simulink model "controller"  (R2017b)
settings: Solver=ode23tb  StartTime=0.0  StopTime=10  RelTol=1e-3
values from neighbouring files (symbols this model uses):
  A = [0 0 1 0 ... (first row only)    [linearizedSS.m]
  B = [0;0;K*v/alpha;-c2*l1*m2/alpha]    [linearizedSS.m]
  C = [1 0 0 0;0 1 0 0]    [linearizedSS.m]
  K = 1.8    [Nonlinearequations.m]    (also in controller.m = place(Phi',Cd',dopoles).'; controllerData2.m = place(Phi',Cd',dopoles).'; linearizedSS.m; pendulumSim.m)
  L = Laug(1:4)    [controller.m]    (also in controllerData2.m)
  x0 = [0.51*pi,0,0.5*pi,0]    [Nonlinearequations.m]    (also in controllerData3.m = [-0.6*pi 0 -0.4*pi 0]; linearizeM.m = [-0.51*pi,0,-0.5*pi,0])
settings Model: Creator=geert  LastModifiedBy=geert

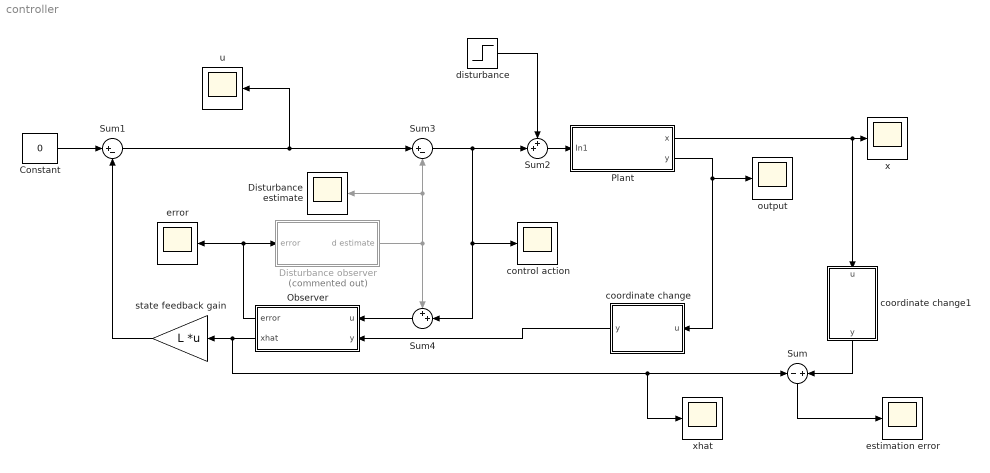
== system controller ==
  Constant : Constant  Value=0
  Disturbance estimate : Scope
  Disturbance observer : Subsystem  Commented=on
  Observer : Subsystem
  Plant : Subsystem
  Sum : Sum  Inputs=-|+
  Sum1 : Sum  Inputs=|+-
  Sum2 : Sum  Inputs=++|
  Sum3 : Sum  Inputs=|+-
  Sum4 : Sum  Inputs=++|
  control action : Scope
  coordinate change : MATLAB Function  TreatAsAtomicUnit=on
  coordinate change1 : MATLAB Function  TreatAsAtomicUnit=on
  disturbance : Step  Time=5  After=0  SampleTime=0
  error : Scope
  estimation error : Scope
  output : Scope
  state feedback gain : Gain  Gain=L  Multiplication=Matrix(K*u)
  u : Scope
  x : Scope
  xhat : Scope
  wires:
  state feedback gain/1 -> Sum1/2
  Sum2/1 -> Plant/1(In1)
  Observer/2(xhat) -> xhat/1, Sum/1, state feedback gain/1
  Sum/1 -> estimation error/1
  disturbance/1 -> Sum2/1
  Sum1/1 -> u/1, Sum3/1
  Constant/1 -> Sum1/1
  Sum4/1 -> Observer/1(u)
  Sum3/1 -> control action/1, Sum4/2, Sum2/2
  Plant/1(x) -> coordinate change1/1(u), x/1
  Plant/2(y) -> coordinate change/1(u), output/1
  Disturbance observer/1(d estimate) -> Disturbance estimate/1, Sum3/2, Sum4/1
  coordinate change/1(y) -> Observer/2(y)
  coordinate change1/1(y) -> Sum/2
  Observer/1(error) -> error/1, Disturbance observer/1(error)

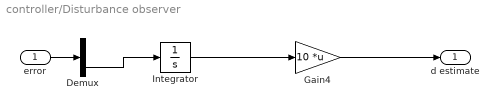
== system controller/Disturbance observer ==
  error : Inport
  Demux : Demux  Outputs=2
  Gain4 : Gain  Gain=10  Multiplication=Matrix(K*u)
  Integrator : Integrator
  d estimate : Outport
  wires:
  Integrator/1 -> Gain4/1
  Gain4/1 -> d estimate/1
  Demux/2 -> Integrator/1
  error/1 -> Demux/1

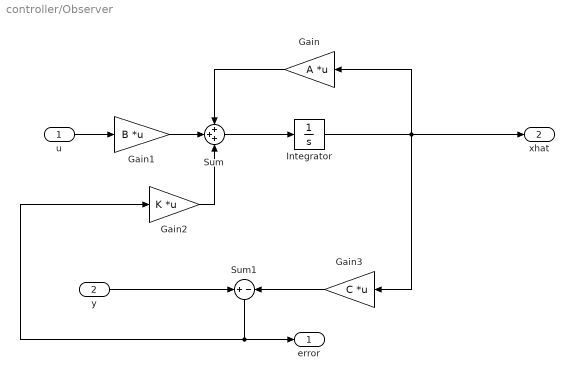
== system controller/Observer ==
  u : Inport
  y : Inport  Port=2
  Gain : Gain  Gain=A  Multiplication=Matrix(K*u)
  Gain1 : Gain  Gain=B  Multiplication=Matrix(K*u)
  Gain2 : Gain  Gain=K  Multiplication=Matrix(K*u)
  Gain3 : Gain  Gain=C  Multiplication=Matrix(K*u)
  Integrator : Integrator  InitialCondition=[0 0 0 0]
  Sum : Sum  Inputs=+++
  Sum1 : Sum  Inputs=+|-
  error : Outport
  xhat : Outport  Port=2
  wires:
  u/1 -> Gain1/1
  Gain1/1 -> Sum/2
  Gain2/1 -> Sum/3
  y/1 -> Sum1/1
  Sum1/1 -> Gain2/1, error/1
  Integrator/1 -> Gain/1, Gain3/1, xhat/1
  Gain3/1 -> Sum1/2
  Gain/1 -> Sum/1
  Sum/1 -> Integrator/1

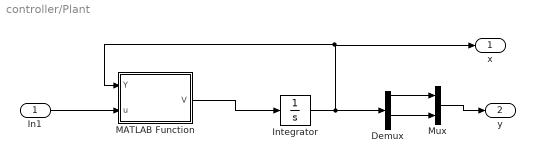
== system controller/Plant ==
  In1 : Inport
  Demux : Demux
  Integrator : Integrator  InitialCondition=x0
  MATLAB Function : MATLAB Function  TreatAsAtomicUnit=on
  Mux : Mux  Inputs=2
  x : Outport
  y : Outport  Port=2
  wires:
  Integrator/1 -> Demux/1, x/1, MATLAB Function/1(Y)
  In1/1 -> MATLAB Function/2(u)
  MATLAB Function/1(V) -> Integrator/1
  Demux/1 -> Mux/1
  Demux/3 -> Mux/2
  Mux/1 -> y/1

== matlab function controller/coordinate change ==
  data: u input; y output
function y = fcn(u)

y = u + 0.5*pi;

== matlab function controller/Plant/MATLAB Function ==
  data: Y input; u input; V output
function V = M(Y,u)
%M
%    V = M(Y,U)

%    This function was generated by the Symbolic Math Toolbox version 8.0.
%    09-May-2018 10:56:52

t3 = Y(1);
t4 = Y(3);
t5 = t3-t4;
t2 = cos(t5);
t6 = t2.^2;
t7 = t6.*7.29e-8;
t8 = t7-8.854411999999999e-6;
t9 = 1.0./t8;
t10 = Y(2);
t11 = Y(4);
t12 = cos(t4);
t13 = cos(t3);
t14 = sin(t5);
t15 = t10.^2;
t16 = t3.*2.0;
t17 = t4.*-2.0+t16;
t18 = sin(t17);
t19 = t11.^2;
V = [t10;t9.*t10.*7.649599999999999e-6+t9.*(t13.*1.013074776e-3-t2.*t12.*4.449816e-5)-t2.*t9.*t11.*9.45e-5+t9.*t14.*t19.*1.032696e-5+t9.*t15.*t18.*3.645000000000001e-8+t2.*t9.*u.*4.86e-4;t11;t9.*(t12.*3.8153052e-5-t2.*t13.*7.15149e-6)+t9.*t11.*8.1025e-5-t9.*u.*4.167e-4-t2.*t9.*t10.*5.4e-8-t9.*t14.*t15.*6.2505e-8-t9.*t18.*t19.*3.645000000000001e-8];

== matlab function controller/coordinate change1 ==
  data: u input; y output
function y = fcn(u)
y = [0 0 0 0];
y(1) = u(1) + 0.5*pi;
y(3) = u(3) + 0.5*pi;
y(2) = u(2);
y(4) = u(4);
